simulink model "Mach1_Multi_Robot_Systems_Project"  (R2024b)
settings: Solver=VariableStepAuto  StartTime=0.0  StopTime=300  RelTol=1e-3
undefined symbols (not defined in the file): sigbuilder_block
libraries: sharedtransform x6, vrlib x6, slpidlib x3, shared6dof x1, aerolibasang x1
(part 2 of 2)

== matlab function Mach1_Multi_Robot_Systems_Project/Plant and Environment model/Propulsion Forces and Moments/Input Command to Thrust/PWM Signals to Thrust/MATLAB Function2 ==
  data: u input; y output
function y = Normalize(u)
y = (u-1500)*150/400;

== matlab function Mach1_Multi_Robot_Systems_Project/Plant and Environment model/Propulsion Forces and Moments/Input Command to Thrust/PWM Signals to Thrust/MATLAB Function3 ==
  data: u input; y output
function y = Normalize(u)
y = (u-1500)*150/400;

== matlab function Mach1_Multi_Robot_Systems_Project/Plant and Environment model/Propulsion Forces and Moments/Input Command to Thrust/PWM Signals to Thrust/MATLAB Function4 ==
  data: u input; y output
function y = Normalize(u)
y = (u-1500)*150/400;

== matlab function Mach1_Multi_Robot_Systems_Project/Plant and Environment model/Dynamics solver/Post-Processing/MATLAB Function ==
  data: Position input; srf_in input
function Visualize(Position, srf_in)

    coder.extrinsic('setax'); 
    setax(Position, srf_in);  

end

== matlab function Mach1_Multi_Robot_Systems_Project/Plant and Environment model/Environmental Forces & Moments/Hydrodynamic Forces - Accurate/Force Exerted due to Drag (Body Axis)/MATLAB Function ==
  data: u input; C_D output
function C_D = Calculate_Drag_Coeff(u)
if u>pi/2
    u = u-pi;
elseif u < -pi/2
    u = u + pi;
end
C_D = 5.25*(u.^2) - 0.315 * (u) + 0.732;
